simulink model "KalmanSimComparison"  (R2017b)
settings: Solver=FixedStepAuto  StartTime=0.0  StopTime=tMax  FixedStep=1  RelTol=1e-3
undefined symbols (not defined in the file): A, B, C, Discrete, R, Time, X0
libraries: ctrlSharedLib x1
settings Model: Creator=daniel  LastModifiedBy=daniel

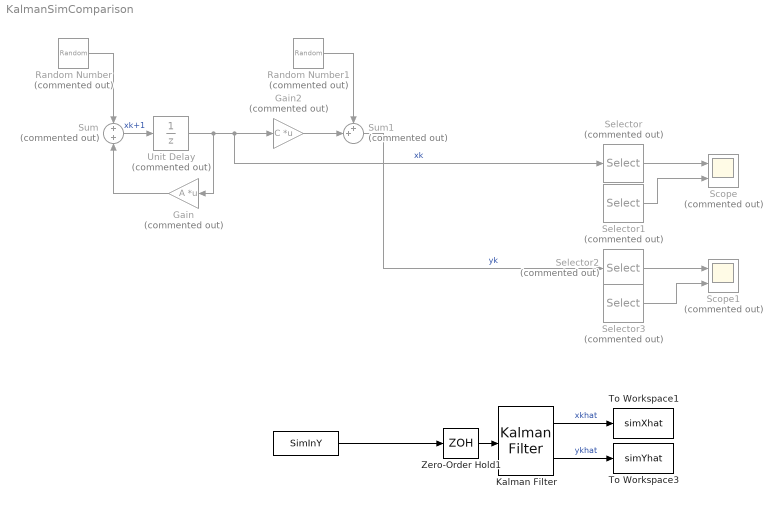
== system KalmanSimComparison ==
  " " : FromWorkspace  VariableName=SimInY  SampleTime=0
  Gain : Gain  Commented=on  Gain=A  Multiplication=Matrix(K*u)
  Gain2 : Gain  Commented=on  Gain=C  Multiplication=Matrix(K*u)
  Kalman Filter : ctrlSharedLib/Kalman Filter  TimeDomain=Discrete-Time  UseCurrentEstimator=on  ModelSource=Individual A, B, C, D matrices  ModelSourceVariable=ss(0.95,1,1,0,1)  A=A  B=B  C=C  D=0  NumberOfStates=1  NumberOfInputs=1  NumberOfOutputs=1  InitialEstimateSource=Dialog  X0=0  P0=10  UseK=off  UseGH=off  NumberOfProcessNoiseInputs=1  G=1  TimeInvariantG=on  H=0  TimeInvariantH=on  Q=Q  TimeInvariantQ=on  R=R  TimeInvariantR=on  N=0  TimeInvariantN=on  AddInputPort=off  AddEnablePort=off  OutputEstimatedY=on  OutputP=off  Ts=-1
      settings: SourceProductBaseCode=CT
  Random Number : RandomNumber  Commented=on  Seed=1234  SampleTime=1
  Random Number1 : RandomNumber  Commented=on  Seed=87654  SampleTime=1
  Scope : Scope  Commented=on  NumInputPorts=2
  Scope1 : Scope  Commented=on  NumInputPorts=2
  Selector : Selector  Commented=on  InputPortWidth=nd  IndexOptions=Index vector (dialog)  Indices=1  OutputSizes=1
  Selector1 : Selector  Commented=on  InputPortWidth=nd  IndexOptions=Index vector (dialog)  Indices=1  OutputSizes=1
  Selector2 : Selector  Commented=on  InputPortWidth=p  IndexOptions=Index vector (dialog)  Indices=1  OutputSizes=1
  Selector3 : Selector  Commented=on  InputPortWidth=p  IndexOptions=Index vector (dialog)  Indices=1  OutputSizes=1
  Sum : Sum  Commented=on
  Sum1 : Sum  Commented=on  Inputs=++|
  To Workspace1 : ToWorkspace  VariableName=simXhat  SaveFormat=Structure With Time  SampleTime=-1
  To Workspace3 : ToWorkspace  VariableName=simYhat  SaveFormat=Structure With Time  SampleTime=-1
  Unit Delay : UnitDelay  Commented=on  InitialCondition=X0  SampleTime=-1
  Zero-Order Hold1 : ZeroOrderHold  SampleTime=-1
  wires:
  Zero-Order Hold1/1 -> Kalman Filter/1
  Kalman Filter/2 -> To Workspace3/1  "ykhat"
  Kalman Filter/1 -> To Workspace1/1  "xkhat"
  Gain/1 -> Sum/2
  Sum1/1 -> Selector2/1  "yk"
  Unit Delay/1 -> Gain/1, Selector/1, Gain2/1  "xk"
  Gain2/1 -> Sum1/2
  Sum/1 -> Unit Delay/1  "xk+1"
  Random Number/1 -> Sum/1
  Random Number1/1 -> Sum1/1
  " "/1 -> Zero-Order Hold1/1
  Selector/1 -> Scope/1
  Selector1/1 -> Scope/2
  Selector2/1 -> Scope1/1
  Selector3/1 -> Scope1/2
